simulink model "bouncing_ball"  (Simulink 8.2)
settings: Solver=ode45  StartTime=0.0  StopTime=10  RelTol=1e-3
libraries: vrlib x2
settings Model: Creator=smahapat  LastModifiedBy=Deepak
settings DebuggingCC: StrictBusMsg=Warning
settings SFSimCC: SimParseCustomCode=off

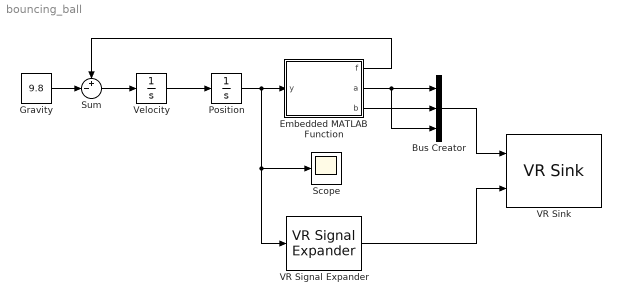
== system bouncing_ball ==
  Bus Creator : BusCreator  Inputs=3
  Embedded MATLAB Function : MATLAB Function  TreatAsAtomicUnit=on
  Gravity : Constant  Value=9.8
  Position : Integrator  InitialCondition=20
  Scope : Scope
      settings: YMin=0  YMax=22.5
  Sum : Sum  Inputs=+-|
  VR Signal Expander : vrlib/VR Signal Expander  outwidth=3  outidx=[2]
  VR Sink : vrlib/VR Sink  InstantiateOnLoad=on  SampleTime=0.01  ViewEnable=on  RemoteChange=off  RemoteView=on  FieldsWritten=Ball.scale.3.1.double#Ball.translation.3.1.double  WorldFileName=bouncing_ball.wrl  AutoView=off  VideoDimensions=[]  AllowVariableSize=off  FigureProperties="{'Position', 'Name', 'Viewpoint', 'CameraBound', 'CameraDirection', 'CameraPosition', 'CameraUpVector', 'ZoomFactor', 'Antialiasing', 'Headlight', 'Lighting', 'NavPanel', 'StatusBar', 'ToolBar', 'Textures', 'Transparency', 'Triad', 'Wireframe', 'NavZones', 'NavMode', 'NavSpeed', 'CaptureFileFormat', 'CaptureFileName', 'Record2DCompressMethod', 'Record2DCompressQuality', 'Record2D', 'Record2DFileName', 'Record2DFPS'; [5.0000000000000000e+00   9.4000000000000000e+01   5.7600000000000000e+02   3.8000000000000000e+02], '', 'My_View', 'on', [0.0000000000000000e+00   0.0000000000000000e+00  -1.0000000000000000e+00], [0.0000000000000000e+00   0.0000000000000000e+00   0.0000000000000000e+00], [0.0000000000000000e+00   1.0000000000000000e+00   0.0000000000000000e+00], [1.0000000000000000e+00], 'on', 'on', 'on', 'halfbar', 'on', 'on', 'on', 'on', 'none', 'off', 'off', 'fly', 'normal', 'tif', '%f_anim_%n.tif', 'auto', [7.5000000000000000e+01], 'off', '%f_anim_%n.avi', [1.5000000000000000e+01]}"
  Velocity : Integrator
  wires:
  Velocity/1 -> Position/1
  Position/1 -> Embedded MATLAB Function/1(y), VR Signal Expander/1, Scope/1
  Sum/1 -> Velocity/1
  VR Signal Expander/1 -> VR Sink/2
  Bus Creator/1 -> VR Sink/1
  Embedded MATLAB Function/3(b) -> Bus Creator/2
  Embedded MATLAB Function/2(a) -> Bus Creator/1, Bus Creator/3
  Embedded MATLAB Function/1(f) -> Sum/1
  Gravity/1 -> Sum/2

== matlab function Embedded MATLAB Function ==
  data: f output double; a output double; b output double; y input double
function [f,a, b] = fcn(y)
%

if y<1e-4
    y=1e-4;
end

if y<1.5
    f=500*(1.5-y);
    a=sqrt(1.5^3/y);
    b=y;
else
    f=0;
    a=1.5;
    b=1.5;
end
